simulink library "Library_Betriebsstrategie"  (R2018b)
settings: Solver=VariableStepAuto  StartTime=0.0  StopTime=10.0  RelTol=1e-3  EnableMultiTasking=on
undefined symbols (not defined in the file): akt_eUELG_HA, akt_eUELG_VA, akt_keinMVS_HA, akt_keinMVS_VA, akt_LSD_HA, akt_LSD_VA, akt_mUELG_HA, akt_mUELG_VA, akt_OD_HA, akt_OD_VA, DiscIntNeverNeededParam, magnitude, mu_road, mu_road_LF, mu_road_LR, mu_road_RF, mu_road_RR, par_MDT, par_VEH, stepsize
libraries: simulink x13
(part 3 of 6)

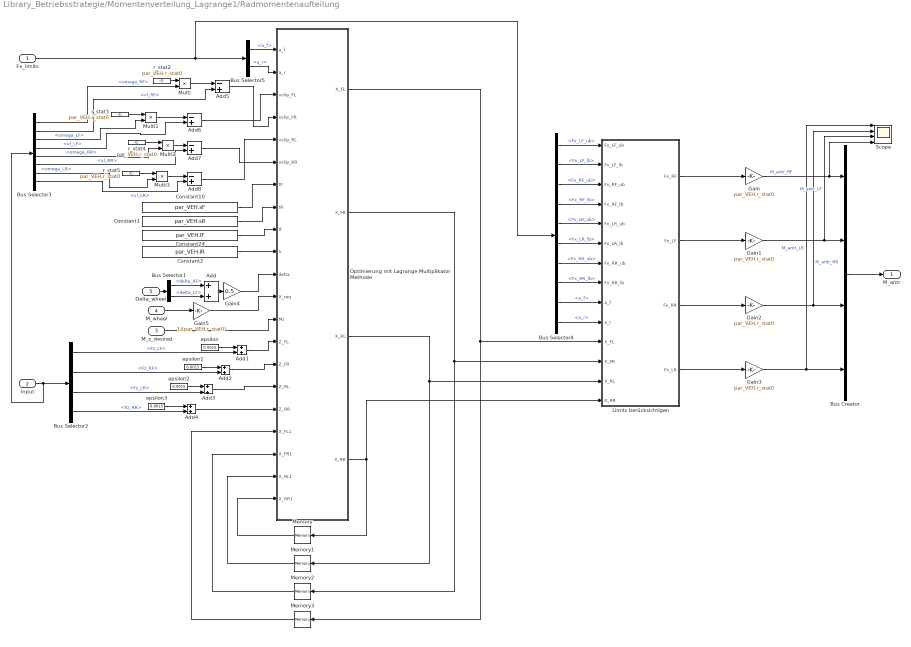
== system Library_Betriebsstrategie/Momentenverteilung_Lagrange1/Radmomentenaufteilung ==
  Fx_limits : Inport
  Input : Inport  Port=2
  M_z_desired : Inport  Port=3
  M_wheel : Inport  Port=4
  Delta_wheel : Inport  Port=5
  Add{,1..4} (5 alike) : Sum
  Add{5..8} (4 alike) : Sum  Inputs=-+
  Bus Creator : BusCreator  Inputs=4
  Bus Selector1 : BusSelector  OutputSignals=delta_RF,delta_LF
  Bus Selector2 : BusSelector  OutputSignals=Fz.Fz_LF,Fz.Fz_RF,Fz.Fz_LR,Fz.Fz_RR
  Bus Selector3 : BusSelector  OutputSignals=omega.omega_RF,vl.vl_RF,omega.omega_LF,vl.vl_LF,omega.omega_RR,vl.vl_RR,omega.omega_LR,vl.vl_LR
  Bus Selector4 : BusSelector  OutputSignals=Fx_LF_ub,Fx_LF_lb,Fx_RF_ub,Fx_RF_lb,Fx_LR_ub,Fx_LR_lb,Fx_RR_ub,Fx_RR_lb,a_f,a_r
  Bus Selector5 : BusSelector  OutputSignals=a_f,a_r
  Constant1 : Constant  Value=par_VEH.sR
  Constant10 : Constant  Value=par_VEH.sF
  Constant2 : Constant  Value=par_VEH.lR
  Constant24 : Constant  Value=par_VEH.lF
  Gain{,1..3} (4 alike) : Gain  Gain=par_VEH.r_stat0
  Gain4 : Gain  Gain=0.5
  Gain5 : Gain  Gain=1/(par_VEH.r_stat0)
  Limits berücksichtigen : MATLAB Function  TreatAsAtomicUnit=on
  Memory{,1..3} (4 alike) : Memory
  Multi{,1..3} (4 alike) : Product  Inputs=**
  Optimierung mit Lagrange Multiplikator Methode : MATLAB Function  TreatAsAtomicUnit=on
  Scope : Scope  NumInputPorts=4
  epsilon{,1..3} (4 alike) : Constant  Value=0.0015
  r_stat{2..5} (4 alike) : Constant  Value=par_VEH.r_stat0
  M_antr : Outport
  wires:
  Bus Selector5/2 -> Optimierung mit Lagrange Multiplikator Methode/2(a_r)  "<a_r>"
  Bus Selector5/1 -> Optimierung mit Lagrange Multiplikator Methode/1(a_f)  "<a_f>"
  Fx_limits/1 -> Bus Selector5/1, Bus Selector4/1
  Limits berücksichtigen/4(Fx_LR) -> Gain3/1
  Limits berücksichtigen/3(Fx_RR) -> Gain2/1
  Limits berücksichtigen/2(Fx_LF) -> Gain1/1
  Limits berücksichtigen/1(Fx_RF) -> Gain/1
  Optimierung mit Lagrange Multiplikator Methode/3(X_RL) -> Memory1/1, Limits berücksichtigen/13(X_RL)
  Bus Selector4/10 -> Limits berücksichtigen/10(a_r)  "<a_r>"
  Bus Selector4/9 -> Limits berücksichtigen/9(a_f)  "<a_f>"
  Bus Selector4/8 -> Limits berücksichtigen/8(Fx_RR_lb)  "<Fx_RR_lb>"
  Bus Selector4/7 -> Limits berücksichtigen/7(Fx_RR_ub)  "<Fx_RR_ub>"
  Bus Selector4/6 -> Limits berücksichtigen/6(Fx_LR_lb)  "<Fx_LR_lb>"
  Bus Selector4/5 -> Limits berücksichtigen/5(Fx_LR_ub)  "<Fx_LR_ub>"
  Bus Selector4/4 -> Limits berücksichtigen/4(Fx_RF_lb)  "<Fx_RF_lb>"
  Bus Selector4/3 -> Limits berücksichtigen/3(Fx_RF_ub)  "<Fx_RF_ub>"
  Bus Selector4/2 -> Limits berücksichtigen/2(Fx_LF_lb)  "<Fx_LF_lb>"
  Bus Selector4/1 -> Limits berücksichtigen/1(Fx_LF_ub)  "<Fx_LF_ub>"
  Memory1/1 -> Optimierung mit Lagrange Multiplikator Methode/20(X_RL1)
  Add3/1 -> Optimierung mit Lagrange Multiplikator Methode/16(Z_RL)
  Bus Creator/1 -> M_antr/1
  Gain/1 -> Scope/4, Bus Creator/1  "M_antr_RF"
  Gain1/1 -> Bus Creator/2, Scope/3  "M_antr_LF"
  Gain2/1 -> Bus Creator/3, Scope/2  "M_antr_RR"
  Gain3/1 -> Bus Creator/4, Scope/1  "M_antr_LR"
  Constant10/1 -> Optimierung mit Lagrange Multiplikator Methode/7(tF)
  Constant1/1 -> Optimierung mit Lagrange Multiplikator Methode/8(tR)
  Constant24/1 -> Optimierung mit Lagrange Multiplikator Methode/9(lf)
  Constant2/1 -> Optimierung mit Lagrange Multiplikator Methode/10(lr)
  Delta_wheel/1 -> Bus Selector1/1
  Bus Selector1/1 -> Add/1  "<delta_RF>"
  Bus Selector1/2 -> Add/2  "<delta_LF>"
  Add/1 -> Gain4/1
  Gain4/1 -> Optimierung mit Lagrange Multiplikator Methode/11(delta)
  M_z_desired/1 -> Optimierung mit Lagrange Multiplikator Methode/13(Mz)
  M_wheel/1 -> Gain5/1
  Gain5/1 -> Optimierung mit Lagrange Multiplikator Methode/12(X_req)
  Optimierung mit Lagrange Multiplikator Methode/1(X_FL) -> Memory3/1, Limits berücksichtigen/11(X_FL)
  Optimierung mit Lagrange Multiplikator Methode/2(X_FR) -> Memory2/1, Limits berücksichtigen/12(X_FR)
  Optimierung mit Lagrange Multiplikator Methode/4(X_RR) -> Memory/1, Limits berücksichtigen/14(X_RR)
  Memory/1 -> Optimierung mit Lagrange Multiplikator Methode/21(X_RR1)
  Memory2/1 -> Optimierung mit Lagrange Multiplikator Methode/19(X_FR1)
  Memory3/1 -> Optimierung mit Lagrange Multiplikator Methode/18(X_FL1)
  Add1/1 -> Optimierung mit Lagrange Multiplikator Methode/14(Z_FL)
  Bus Selector2/4 -> Add4/2  "<Fz_RR>"
  Bus Selector2/3 -> Add3/2  "<Fz_LR>"
  Bus Selector2/2 -> Add2/2  "<Fz_RF>"
  Bus Selector2/1 -> Add1/2  "<Fz_LF>"
  Add4/1 -> Optimierung mit Lagrange Multiplikator Methode/17(Z_RR)
  Add2/1 -> Optimierung mit Lagrange Multiplikator Methode/15(Z_FR)
  epsilon/1 -> Add1/1
  epsilon1/1 -> Add2/1
  epsilon2/1 -> Add3/1
  epsilon3/1 -> Add4/1
  Add7/1 -> Optimierung mit Lagrange Multiplikator Methode/6(vslip_RR)
  Add8/1 -> Optimierung mit Lagrange Multiplikator Methode/5(vslip_RL)
  Bus Selector3/8 -> Add8/2  "<vl_LR>"
  Bus Selector3/6 -> Add7/2  "<vl_RR>"
  Bus Selector3/4 -> Add6/2  "<vl_LF>"
  Bus Selector3/7 -> Multi3/2  "<omega_LR>"
  Bus Selector3/5 -> Multi2/2  "<omega_RR>"
  Bus Selector3/3 -> Multi1/2  "<omega_LF>"
  Multi2/1 -> Add7/1
  Multi3/1 -> Add8/1
  r_stat5/1 -> Multi3/1
  r_stat4/1 -> Multi2/1
  Multi1/1 -> Add6/1
  r_stat3/1 -> Multi1/1
  Bus Selector3/2 -> Add5/2  "<vl_RF>"
  Multi/1 -> Add5/1
  Bus Selector3/1 -> Multi/2  "<omega_RF>"
  Input/1 -> Bus Selector3/1, Bus Selector2/1
  Add5/1 -> Optimierung mit Lagrange Multiplikator Methode/4(vslip_FR)
  Add6/1 -> Optimierung mit Lagrange Multiplikator Methode/3(vslip_FL)
  r_stat2/1 -> Multi/1

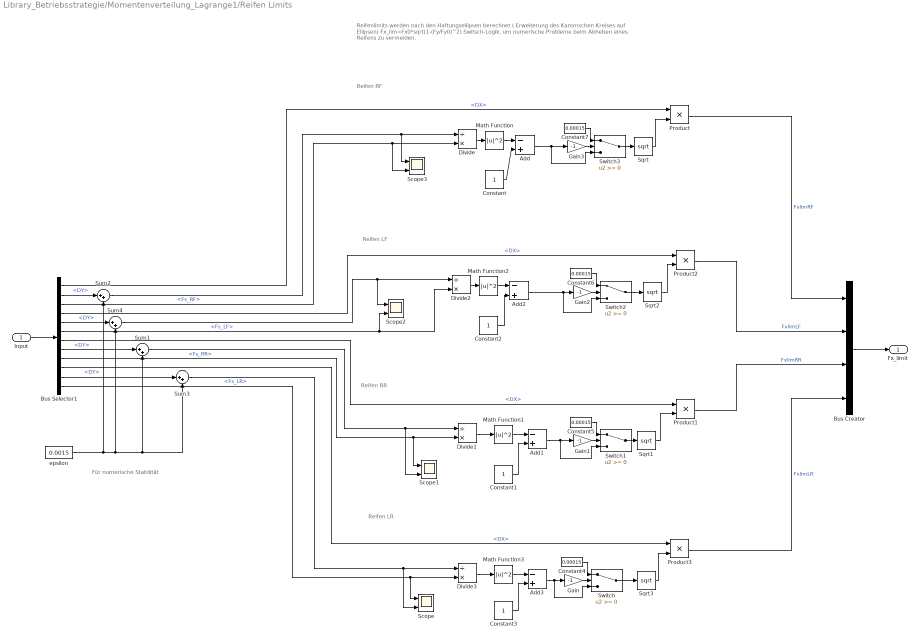
== system Library_Betriebsstrategie/Momentenverteilung_Lagrange1/Reifen Limits ==
  note: Reifen RF
  note: Reifen LF
  note: Reifen RR
  note: Reifen LR
  note: Für numerische Stabilität
  note: Reifenlimits werden nach den Haftungsellipsen berechnet ( Erweiterung des Kammschen Kreises auf Ellipsen)
      | Fx_lim=Fx0*sqrt(1-(Fy/Fy0)^2)
      |
      | Switsch-Logik, um numerische Probleme beim Abheben eines Reifens zu vermeiden.
  Input : Inport
  Add{,1..3} (4 alike) : Sum  Inputs=-+
  Bus Creator : BusCreator  Inputs=4
  Bus Selector1 : BusSelector  OutputSignals=F0.F0_RF.DX,F0.F0_RF.DY,Fs.Fs_RF,F0.F0_LF.DX,F0.F0_LF.DY,Fs.Fs_LF,F0.F0_RR.DX,F0.F0_RR.DY,Fs.Fs_RR,F0.F0_LR.DX,F0.F0_LR.DY,Fs.Fs_LR
  Constant{,1..3} (4 alike) : Constant
  Constant{4..7} (4 alike) : Constant  Value=0.00015
  Divide{,1..3} (4 alike) : Product  Inputs=/*
  Gain{,1..3} (4 alike) : Gain  Gain=-1
  Math Function{,1..3} (4 alike) : Math  Operator=magnitude^2  SaturateOnIntegerOverflow=on
  Product{,1..3} (4 alike) : Product
  Scope{,1..3} (4 alike) : Scope  NumInputPorts=2
  Sqrt{,1..3} (4 alike) : Sqrt  SaturateOnIntegerOverflow=on
  Sum{1..4} (4 alike) : Sum  Inputs=|++
  Switch{,1..3} (4 alike) : Switch
  epsilon : Constant  Value=0.0015
  Fx_limit : Outport
  wires:
  Bus Selector1/10 -> Product3/1  "<DX>"
  Bus Selector1/5 -> Sum4/1  "<DY>"
  Bus Selector1/8 -> Sum1/1  "<DY>"
  Bus Selector1/11 -> Sum3/1  "<DY>"
  Bus Selector1/2 -> Sum2/1  "<DY>"
  epsilon/1 -> Sum3/2, Sum1/2, Sum4/2, Sum2/2
  Bus Selector1/1 -> Product/1  "<DX>"
  Sum2/1 -> Divide/1, Scope3/1
  Math Function/1 -> Add/1
  Constant/1 -> Add/2
  Sqrt/1 -> Product/2
  Bus Selector1/7 -> Product1/1  "<DX>"
  Sum1/1 -> Divide1/1, Scope1/2
  Divide1/1 -> Math Function1/1
  Math Function1/1 -> Add1/1
  Constant1/1 -> Add1/2
  Sqrt1/1 -> Product1/2
  Bus Selector1/4 -> Product2/1  "<DX>"
  Sum4/1 -> Divide2/1, Scope2/1
  Divide2/1 -> Math Function2/1
  Math Function2/1 -> Add2/1
  Constant2/1 -> Add2/2
  Sqrt2/1 -> Product2/2
  Sum3/1 -> Divide3/1, Scope/2
  Divide3/1 -> Math Function3/1
  Math Function3/1 -> Add3/1
  Constant3/1 -> Add3/2
  Sqrt3/1 -> Product3/2
  Divide/1 -> Math Function/1
  Input/1 -> Bus Selector1/1
  Bus Selector1/3 -> Divide/2, Scope3/2  "<Fs_RF>"
  Bus Selector1/6 -> Divide2/2, Scope2/2  "<Fs_LF>"
  Bus Selector1/9 -> Divide1/2, Scope1/1  "<Fs_RR>"
  Bus Selector1/12 -> Divide3/2, Scope/1  "<Fs_LR>"
  Product/1 -> Bus Creator/1  "FxlimRF"
  Product2/1 -> Bus Creator/2  "FxlimLF"
  Product1/1 -> Bus Creator/3  "FxlimRR"
  Product3/1 -> Bus Creator/4  "FxlimLR"
  Bus Creator/1 -> Fx_limit/1
  Add3/1 -> Switch/3, Gain/1
  Gain/1 -> Switch/2
  Constant4/1 -> Switch/1
  Switch/1 -> Sqrt3/1
  Add1/1 -> Gain1/1, Switch1/3
  Gain1/1 -> Switch1/2
  Constant5/1 -> Switch1/1
  Switch1/1 -> Sqrt1/1
  Add2/1 -> Switch2/3, Gain2/1
  Gain2/1 -> Switch2/2
  Constant6/1 -> Switch2/1
  Switch2/1 -> Sqrt2/1
  Add/1 -> Gain3/1, Switch3/3
  Gain3/1 -> Switch3/2
  Constant7/1 -> Switch3/1
  Switch3/1 -> Sqrt/1

== system Library_Betriebsstrategie/Momentenverteilung_Lagrange2/Feedback Controller ==
  note: 1/2 sigma(Tc)
  note: M_z punkt = - Iz * K * sign(sigma - 1/2sigma(Tc))
  note: Sigmoid Funktion
  Input : Inport
  Gierrate ref : Inport  Port=2
  -1 : Gain  Gain=-1
  Abs : Abs
  Add : Sum
  Bus Selector2 : BusSelector  OutputSignals=psi.psip
  Constant1 : Constant  Value=par_VEH.Iz
  Discrete D : simulink/Discrete/Discrete Derivative  gainval=1.0  ICPrevScaledInput=0.0  OutMin=[]  OutMax=[]  OutDataType=fixdt(1, 16)  OutScaling=2^-10  DoSatur=off
  Discrete-Time Integrator : DiscreteIntegrator  SampleTime=-1  LimitOutput=on  UpperSaturationLimit=par_VEH.Iz/10  LowerSaturationLimit=-par_VEH.Iz/10  ICPrevOutput=DiscIntNeverNeededParam  ICPrevScaledInput=DiscIntNeverNeededParam
  Divide : Product  Inputs=*/
  Divide1 : Product  Inputs=*/
  Einheitenkorrektur : Constant  Value=1000
  Gain : Gain  Gain=0.5
  K : Gain  Gain=8
  Memory : Memory  LinearizeAsDelay=on
  Product : Product
  Scope : Scope  NumInputPorts=2
  Sum : Sum  Inputs=|-+
  Sum1 : Sum  Inputs=|+-
  Unit Delay : UnitDelay  SampleTime=-1
  Zero Crossing : Subsystem
  epsilon : Constant  Value=0.015
  M_z_desired : Outport
  wires:
  Gierrate ref/1 -> Scope/1, Sum/1
  Sum/1 -> Sum1/1, Zero Crossing/3(e0), Discrete D/1  "sigma = - error"
  Sum1/1 -> Divide/1, Abs/1
  Abs/1 -> Add/1
  epsilon/1 -> Add/2
  Add/1 -> Divide/2
  Divide/1 -> K/1
  K/1 -> Product/1
  Product/1 -> -1/1
  -1/1 -> Discrete-Time Integrator/1
  Discrete-Time Integrator/1 -> M_z_desired/1
  Discrete D/1 -> Zero Crossing/1(de0), Unit Delay/1
  Gain/1 -> Sum1/2
  Memory/1 -> Zero Crossing/4(e1)
  Unit Delay/1 -> Zero Crossing/2(de1)
  Zero Crossing/1(error(Tc)) -> Memory/1, Gain/1
  Einheitenkorrektur/1 -> Divide1/2
  Divide1/1 -> Product/2
  Input/1 -> Bus Selector2/1
  Bus Selector2/1 -> Scope/2, Sum/2  "<psip>"
  Constant1/1 -> Divide1/1

== system Library_Betriebsstrategie/Momentenverteilung_Lagrange2/Gierrate Referenz Berechnung ==
  note: Gewünschte Gierrate nach:
      | psip_desired = vx * delta / (l + vx^2 * K_us )
  note: Limit für die Gierrate
  input : Inport
  delta_wheel : Inport  Port=2
  2 Räder : Constant  Value=0.5
  Abs : Abs
  Abs1 : Abs
  Add : Sum
  Add1 : Sum  Inputs=+--
  Add2 : Sum
  Bus Selector1 : BusSelector  OutputSignals=delta_RF,delta_LF
  Bus Selector2 : BusSelector  OutputSignals=x.ax,beta.beta,beta.betap,x.vx
  Constant1 : Constant  Value=par_VEH.g
  Constant10 : Constant  Value=par_VEH.l
  Constant20 : Constant  Value=0.25*(mu_road_RF+mu_road_RR+mu_road_LF+mu_road_LR)
  Divide : Product  Inputs=*/
  Divide1 : Product  Inputs=**/
  Divide2 : Product  Inputs=**/
  Divide3 : Product  Inputs=*/
  Kus : Constant  Value=0
  Product : Product
  Product1 : Product
  Product2 : Product
  Scope : Scope  NumInputPorts=2
  Sicherheitsfaktor : Gain  Gain=0.90
  Sign : Signum
  Sqrt : Sqrt  SaturateOnIntegerOverflow=on
  Sum : Sum  Inputs=|++
  Sum1 : Sum  Inputs=|++
  delta mittel : Product
  eins : Constant
  epsilon : Constant  Value=0.0015
  min : MinMax  Inputs=2
  tan (beta)1 : Trigonometry  Operator=tan
  tan^2 (beta)1 : Math  Operator=square  SaturateOnIntegerOverflow=on
  vx^2 : Math  Operator=square  SaturateOnIntegerOverflow=on
  Gierrate ref : Outport
  wires:
  Product/1 -> Divide/1
  Constant10/1 -> Sum/2
  vx^2/1 -> Product1/1
  Sum/1 -> Divide/2
  Product1/1 -> Sum/1
  Kus/1 -> Product1/2
  Divide/1 -> Abs/1  "Gierrate gewuenscht"
  delta_wheel/1 -> Bus Selector1/1
  Bus Selector1/1 -> Add/1  "<delta_RF>"
  Bus Selector1/2 -> Add/2  "<delta_LF>"
  Add/1 -> Scope/2, delta mittel/1
  2 Räder/1 -> delta mittel/2
  delta mittel/1 -> Sign/1, Product/2
  input/1 -> Bus Selector2/1
  Bus Selector2/4 -> Sum1/1, vx^2/1, Product/1  "<vx>"
  Sicherheitsfaktor/1 -> Abs1/1  "Gierrate Limit"
  Add1/1 -> Sicherheitsfaktor/1
  Sign/1 -> Product2/1  "Vorzeichen von delta"
  min/1 -> Product2/2
  Product2/1 -> Scope/1, Gierrate ref/1
  Abs/1 -> min/1
  Abs1/1 -> min/2
  Divide1/1 -> Add1/1
  Constant1/1 -> Divide1/2
  Constant20/1 -> Divide1/1
  Divide2/1 -> Add1/2
  Bus Selector2/1 -> Divide2/2  "<ax>"
  tan (beta)1/1 -> tan^2 (beta)1/1, Divide2/1
  Bus Selector2/2 -> tan (beta)1/1  "<beta>"
  Divide3/1 -> Add1/3
  Bus Selector2/3 -> Divide3/1  "<betap>"
  tan^2 (beta)1/1 -> Add2/1
  eins/1 -> Add2/2
  Add2/1 -> Sqrt/1
  Sqrt/1 -> Divide3/2
  Sum1/1 -> Divide2/3, Divide1/3
  epsilon/1 -> Sum1/2

== system Library_Betriebsstrategie/Momentenverteilung_Lagrange2/Limitierungen gesamt (mit MVS Limits) ==
  Fx_limit : Inport
  M_limit : Inport  Port=2
  M_limit_zentral : Inport  Port=3
  Aktuatoren und Delta TV : Subsystem
  Bus Creator : BusCreator  Inputs=10
  Bus Selector : BusSelector  OutputSignals=FxlimRF,FxlimLF,FxlimRR,FxlimLR
  Bus Selector1 : BusSelector  OutputSignals=M_RF_ub,M_RF_lb,M_LF_ub,M_LF_lb,M_RR_ub,M_RR_lb,M_LR_ub,M_LR_lb
  Bus Selector2 : BusSelector  OutputSignals=M_F_lb,M_F_ub,M_R_lb,M_R_ub
  Limits Zusammenführung : MATLAB Function  TreatAsAtomicUnit=on
  Scope : Scope  NumInputPorts=4
  Scope1 : Scope  NumInputPorts=4
  Scope2 : Scope  NumInputPorts=4
  r_stat0 : Constant  Value=par_VEH.r_stat0
  Fx_limits : Outport
  wires:
  Limits Zusammenführung/8(Fx_RR_lb) -> Bus Creator/8  "Fx_RR_lb"
  Limits Zusammenführung/7(Fx_RR_ub) -> Bus Creator/7  "Fx_RR_ub"
  Limits Zusammenführung/6(Fx_LR_lb) -> Bus Creator/6  "Fx_LR_lb"
  Limits Zusammenführung/5(Fx_LR_ub) -> Bus Creator/5  "Fx_LR_ub"
  Limits Zusammenführung/4(Fx_RF_lb) -> Bus Creator/4, Scope1/1  "Fx_RF_lb"
  Limits Zusammenführung/3(Fx_RF_ub) -> Bus Creator/3, Scope1/2  "Fx_RF_ub"
  Limits Zusammenführung/2(Fx_LF_lb) -> Bus Creator/2, Scope1/3  "Fx_LF_lb"
  Limits Zusammenführung/1(Fx_LF_ub) -> Bus Creator/1, Scope1/4  "Fx_LF_ub"
  Aktuatoren und Delta TV/2(Delta_T_r) -> Scope2/2, Limits Zusammenführung/18(DELTA_T_r)
  Aktuatoren und Delta TV/1(Delta_T_f) -> Scope2/1, Limits Zusammenführung/17(DELTA_T_f)
  r_stat0/1 -> Limits Zusammenführung/21(r)
  Fx_limit/1 -> Bus Selector/1
  M_limit/1 -> Bus Selector1/1
  Bus Creator/1 -> Fx_limits/1
  Bus Selector/1 -> Limits Zusammenführung/1(FxlimRF), Scope/4  "<FxlimRF>"
  Bus Selector/2 -> Limits Zusammenführung/2(FxlimLF), Scope/3  "<FxlimLF>"
  Bus Selector/3 -> Scope/2, Limits Zusammenführung/3(FxlimRR)  "<FxlimRR>"
  Bus Selector/4 -> Limits Zusammenführung/4(FxlimLR), Scope/1  "<FxlimLR>"
  Bus Selector1/1 -> Limits Zusammenführung/5(M_RF_ub)  "<M_RF_ub>"
  Bus Selector1/2 -> Limits Zusammenführung/6(M_RF_lb)  "<M_RF_lb>"
  Bus Selector1/3 -> Limits Zusammenführung/7(M_LF_ub)  "<M_LF_ub>"
  Bus Selector1/4 -> Limits Zusammenführung/8(M_LF_lb)  "<M_LF_lb>"
  Bus Selector1/5 -> Limits Zusammenführung/9(M_RR_ub)  "<M_RR_ub>"
  Bus Selector1/6 -> Limits Zusammenführung/10(M_RR_lb)  "<M_RR_lb>"
  Bus Selector1/7 -> Limits Zusammenführung/11(M_LR_ub)  "<M_LR_ub>"
  Bus Selector1/8 -> Limits Zusammenführung/12(M_LR_lb)  "<M_LR_lb>"
  M_limit_zentral/1 -> Bus Selector2/1
  Bus Selector2/1 -> Limits Zusammenführung/13(M_F_lb)  "<M_F_lb>"
  Bus Selector2/2 -> Limits Zusammenführung/14(M_F_ub)  "<M_F_ub>"
  Bus Selector2/3 -> Limits Zusammenführung/15(M_R_lb)  "<M_R_lb>"
  Bus Selector2/4 -> Limits Zusammenführung/16(M_R_ub)  "<M_R_ub>"
  Aktuatoren und Delta TV/3(A_f) -> Scope2/3, Bus Creator/9, Limits Zusammenführung/19(a_f)
  Aktuatoren und Delta TV/4(A_r) -> Scope2/4, Bus Creator/10, Limits Zusammenführung/20(a_r)

== system Library_Betriebsstrategie/Momentenverteilung_Lagrange2/Momente für die Reibbremse ==
  M_antr : Inport
  M_wheel : Inport  Port=2
  v_x : Inport  Port=3
  Add : Sum  Inputs=-+
  Add1 : Sum  Inputs=++++
  Bias : Bias  Bias=-1
  Bus Creator1 : BusCreator  Inputs=4
  Bus Selector : BusSelector  OutputSignals=M_antr_LF,M_antr_LR,M_antr_RF,M_antr_RR
  Constant1 : Constant  Value=par_VEH.bkv
  Product4 : Product  Inputs=3
  Product5 : Product  Inputs=3
  Saturation2 : Saturate  UpperLimit=0  LowerLimit=-5000
  Sign : Signum
  Signal Conversion : SignalConversion  OverrideOpt=off
  Signal Conversion1 : SignalConversion  OverrideOpt=off
  Unary Minus : UnaryMinus
  Unit Delay2 : UnitDelay  InitialCondition=2  SampleTime=-1
  M_brems : Outport
  wires:
  Add/1 -> Saturation2/1
  Saturation2/1 -> Product5/1, Product4/2
  Bias/1 -> Unary Minus/1
  Unary Minus/1 -> Product5/2
  Sign/1 -> Product4/3, Product5/3
  Unit Delay2/1 -> Sign/1
  Constant1/1 -> Product4/1, Bias/1
  v_x/1 -> Unit Delay2/1
  M_wheel/1 -> Add/2
  M_antr/1 -> Bus Selector/1
  Bus Selector/4 -> Add1/4  "<M_antr_RR>"
  Bus Selector/3 -> Add1/3  "<M_antr_RF>"
  Bus Selector/2 -> Add1/2  "<M_antr_LR>"
  Bus Selector/1 -> Add1/1  "<M_antr_LF>"
  Add1/1 -> Add/1
  Bus Creator1/1 -> M_brems/1
  Product4/1 -> Bus Creator1/1, Signal Conversion/1  "M_brems_LF"
  Signal Conversion/1 -> Bus Creator1/2  "M_brems_LR"
  Product5/1 -> Signal Conversion1/1, Bus Creator1/3  "M_brems_RF"
  Signal Conversion1/1 -> Bus Creator1/4  "M_brems_RR"

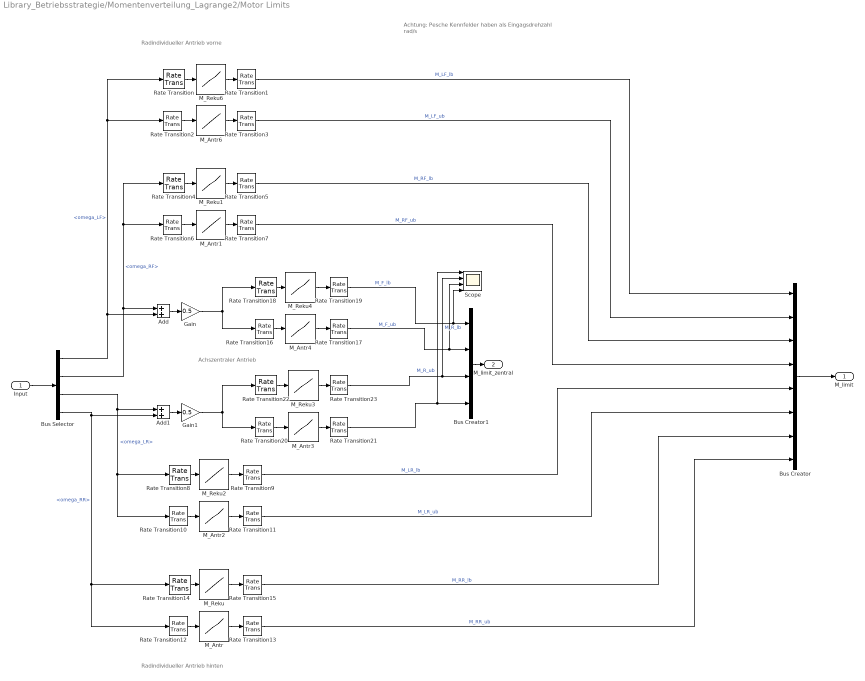
== system Library_Betriebsstrategie/Momentenverteilung_Lagrange2/Motor Limits ==
  note: Achszentraler Antrieb
  note: Radindividueller Antrieb hinten
  note: Radindividueller Antrieb vorne
  note: Achtung:
      | Pesche Kennfelder haben als Eingagsdrehzahl rad/s
  Input : Inport
  Add : Sum
  Add1 : Sum
  Bus Creator : BusCreator  Inputs=8
  Bus Creator1 : BusCreator  Inputs=4
  Bus Selector : BusSelector  OutputSignals=omega.omega_LF,omega.omega_RF,omega.omega_LR,omega.omega_RR
  Gain : Gain  Gain=0.5
  Gain1 : Gain  Gain=0.5
  M_Antr : Lookup_n-D  NumberOfTableDimensions=1  BreakpointsForDimension1=par_MDT.HA.em.MaxMotorTrqCurve_w/par_MDT.HA.trans.i_gears(1)  Table=par_MDT.HA.em.MaxMotorTrqCurve_M*par_MDT.HA.trans.i_gears(1)  ExtrapMethod=Clip  UseLastTableValue=on  InternalRulePriority=Speed  RndMeth=Simplest  InputSameDT=on
  M_Antr1 : Lookup_n-D  NumberOfTableDimensions=1  BreakpointsForDimension1=par_MDT.VA.em.MaxMotorTrqCurve_w/par_MDT.VA.trans.i_gears(1)  Table=par_MDT.VA.em.MaxMotorTrqCurve_M*par_MDT.VA.trans.i_gears(1)  ExtrapMethod=Clip  UseLastTableValue=on  InternalRulePriority=Speed  RndMeth=Simplest  InputSameDT=on
  M_Antr2 : Lookup_n-D  NumberOfTableDimensions=1  BreakpointsForDimension1=par_MDT.HA.em.MaxMotorTrqCurve_w/par_MDT.HA.trans.i_gears(1)  Table=par_MDT.HA.em.MaxMotorTrqCurve_M*par_MDT.HA.trans.i_gears(1)  ExtrapMethod=Clip  UseLastTableValue=on  InternalRulePriority=Speed  RndMeth=Simplest  InputSameDT=on
  M_Antr3 : Lookup_n-D  NumberOfTableDimensions=1  BreakpointsForDimension1=par_MDT.HA.em.MaxMotorTrqCurve_w/par_MDT.HA.trans.i_gears(1)  Table=par_MDT.HA.em.MaxMotorTrqCurve_M*par_MDT.HA.trans.i_gears(1)  ExtrapMethod=Clip  UseLastTableValue=on  InternalRulePriority=Speed  RndMeth=Simplest  InputSameDT=on
  M_Antr4 : Lookup_n-D  NumberOfTableDimensions=1  BreakpointsForDimension1=par_MDT.VA.em.MaxMotorTrqCurve_w/par_MDT.VA.trans.i_gears(1)  Table=par_MDT.VA.em.MaxMotorTrqCurve_M*par_MDT.VA.trans.i_gears(1)  ExtrapMethod=Clip  UseLastTableValue=on  InternalRulePriority=Speed  RndMeth=Simplest  InputSameDT=on
  M_Antr6 : Lookup_n-D  NumberOfTableDimensions=1  BreakpointsForDimension1=par_MDT.VA.em.MaxMotorTrqCurve_w/par_MDT.VA.trans.i_gears(1)  Table=par_MDT.VA.em.MaxMotorTrqCurve_M*par_MDT.VA.trans.i_gears(1)  ExtrapMethod=Clip  UseLastTableValue=on  InternalRulePriority=Speed  RndMeth=Simplest  InputSameDT=on
  M_Reku : Lookup_n-D  NumberOfTableDimensions=1  BreakpointsForDimension1=par_MDT.HA.em.MaxGeneratorTrqCurve_w/par_MDT.HA.trans.i_gears(1)  Table=par_MDT.HA.em.MaxGeneratorTrqCurve_M*par_MDT.HA.trans.i_gears(1)  ExtrapMethod=Clip  UseLastTableValue=on  InternalRulePriority=Speed  RndMeth=Simplest  InputSameDT=on
  M_Reku1 : Lookup_n-D  NumberOfTableDimensions=1  BreakpointsForDimension1=par_MDT.VA.em.MaxGeneratorTrqCurve_w/par_MDT.VA.trans.i_gears(1)  Table=par_MDT.VA.em.MaxGeneratorTrqCurve_M*par_MDT.VA.trans.i_gears(1)  ExtrapMethod=Clip  UseLastTableValue=on  InternalRulePriority=Speed  RndMeth=Simplest  InputSameDT=on
  M_Reku2 : Lookup_n-D  NumberOfTableDimensions=1  BreakpointsForDimension1=par_MDT.HA.em.MaxGeneratorTrqCurve_w/par_MDT.HA.trans.i_gears(1)  Table=par_MDT.HA.em.MaxGeneratorTrqCurve_M*par_MDT.HA.trans.i_gears(1)  ExtrapMethod=Clip  UseLastTableValue=on  InternalRulePriority=Speed  RndMeth=Simplest  InputSameDT=on
  M_Reku3 : Lookup_n-D  NumberOfTableDimensions=1  BreakpointsForDimension1=par_MDT.HA.em.MaxGeneratorTrqCurve_w/par_MDT.HA.trans.i_gears(1)  Table=par_MDT.HA.em.MaxGeneratorTrqCurve_M*par_MDT.HA.trans.i_gears(1)  ExtrapMethod=Clip  UseLastTableValue=on  InternalRulePriority=Speed  RndMeth=Simplest  InputSameDT=on
  M_Reku4 : Lookup_n-D  NumberOfTableDimensions=1  BreakpointsForDimension1=par_MDT.VA.em.MaxGeneratorTrqCurve_w/par_MDT.VA.trans.i_gears(1)  Table=par_MDT.VA.em.MaxGeneratorTrqCurve_M*par_MDT.VA.trans.i_gears(1)  ExtrapMethod=Clip  UseLastTableValue=on  InternalRulePriority=Speed  RndMeth=Simplest  InputSameDT=on
  M_Reku6 : Lookup_n-D  NumberOfTableDimensions=1  BreakpointsForDimension1=par_MDT.VA.em.MaxGeneratorTrqCurve_w/par_MDT.VA.trans.i_gears(1)  Table=par_MDT.VA.em.MaxGeneratorTrqCurve_M*par_MDT.VA.trans.i_gears(1)  ExtrapMethod=Clip  UseLastTableValue=on  InternalRulePriority=Speed  RndMeth=Simplest  InputSameDT=on
  Rate Transition{,2,4,6,8,10,12,14,16,18,20,22} (12 alike) : RateTransition  OutPortSampleTime=stepsize*10
  Rate Transition{1,3,5,7,9,11,13,15,17,19,21,23} (12 alike) : RateTransition  OutPortSampleTimeOpt=Inherit  OutPortSampleTime=0.001
  Scope : Scope  NumInputPorts=4
  M_limit : Outport
  M_limit_zentral : Outport  Port=2
  wires:
  Rate Transition17/1 -> Bus Creator1/2, Scope/3  "M_F_ub"
  Bus Creator1/1 -> M_limit_zentral/1
  Bus Creator/1 -> M_limit/1
  Rate Transition13/1 -> Bus Creator/8  "M_RR_ub"
  Rate Transition15/1 -> Bus Creator/7  "M_RR_lb"
  Rate Transition11/1 -> Bus Creator/6  "M_LR_ub"
  Rate Transition9/1 -> Bus Creator/5  "M_LR_lb"
  Rate Transition1/1 -> Bus Creator/1  "M_LF_lb"
  Rate Transition7/1 -> Bus Creator/4  "M_RF_ub"
  Rate Transition5/1 -> Bus Creator/3  "M_RF_lb"
  Rate Transition3/1 -> Bus Creator/2  "M_LF_ub"
  Input/1 -> Bus Selector/1
  Rate Transition2/1 -> M_Antr6/1
  M_Antr6/1 -> Rate Transition3/1
  M_Reku6/1 -> Rate Transition1/1
  Bus Selector/1 -> Add/2, Rate Transition2/1, Rate Transition/1  "<omega_LF>"
  Rate Transition6/1 -> M_Antr1/1
  M_Antr1/1 -> Rate Transition7/1
  Rate Transition4/1 -> M_Reku1/1
  M_Reku1/1 -> Rate Transition5/1
  Bus Selector/2 -> Rate Transition6/1, Rate Transition4/1, Add/1  "<omega_RF>"
  Rate Transition10/1 -> M_Antr2/1
  M_Antr2/1 -> Rate Transition11/1
  Rate Transition8/1 -> M_Reku2/1
  M_Reku2/1 -> Rate Transition9/1
  Rate Transition12/1 -> M_Antr/1
  M_Antr/1 -> Rate Transition13/1
  Rate Transition14/1 -> M_Reku/1
  M_Reku/1 -> Rate Transition15/1
  Bus Selector/3 -> Add1/1, Rate Transition8/1, Rate Transition10/1  "<omega_LR>"
  Bus Selector/4 -> Add1/2, Rate Transition12/1, Rate Transition14/1  "<omega_RR>"
  Rate Transition16/1 -> M_Antr4/1
  M_Antr4/1 -> Rate Transition17/1
  Rate Transition18/1 -> M_Reku4/1
  M_Reku4/1 -> Rate Transition19/1
  Rate Transition20/1 -> M_Antr3/1
  M_Antr3/1 -> Rate Transition21/1
  Rate Transition22/1 -> M_Reku3/1
  M_Reku3/1 -> Rate Transition23/1
  Add/1 -> Gain/1
  Gain/1 -> Rate Transition16/1, Rate Transition18/1
  Add1/1 -> Gain1/1
  Gain1/1 -> Rate Transition20/1, Rate Transition22/1
  Rate Transition19/1 -> Bus Creator1/1, Scope/4  "M_F_lb"
  Rate Transition23/1 -> Bus Creator1/3, Scope/2  "M_R_lb"
  Rate Transition21/1 -> Bus Creator1/4, Scope/1  "M_R_ub"
  Rate Transition/1 -> M_Reku6/1

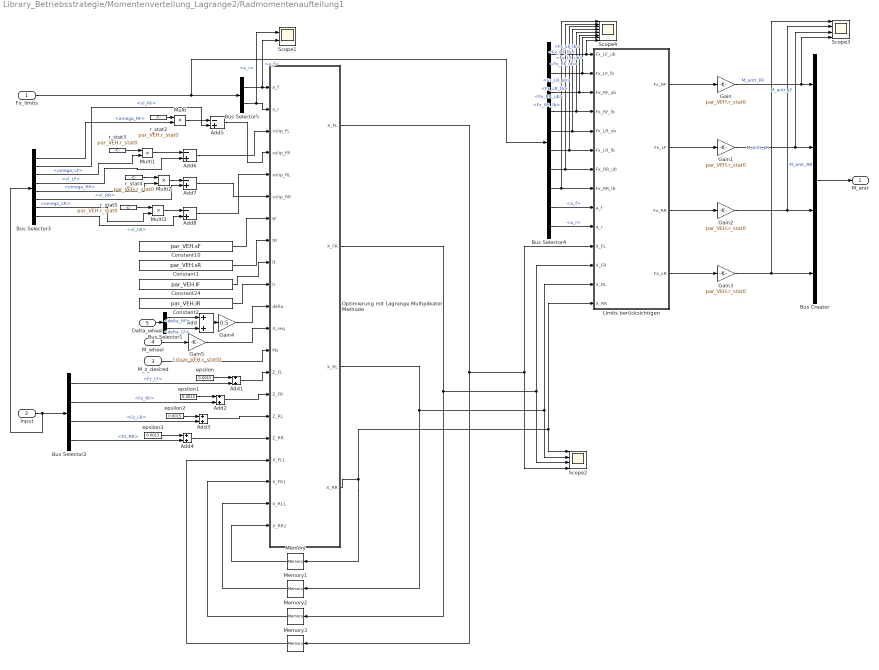
== system Library_Betriebsstrategie/Momentenverteilung_Lagrange2/Radmomentenaufteilung1 ==
  Fx_limits : Inport
  Input : Inport  Port=2
  M_z_desired : Inport  Port=3
  M_wheel : Inport  Port=4
  Delta_wheel : Inport  Port=5
  Add{,1..4} (5 alike) : Sum
  Add{5..8} (4 alike) : Sum  Inputs=-+
  Bus Creator : BusCreator  Inputs=4
  Bus Selector1 : BusSelector  OutputSignals=delta_RF,delta_LF
  Bus Selector2 : BusSelector  OutputSignals=Fz.Fz_LF,Fz.Fz_RF,Fz.Fz_LR,Fz.Fz_RR
  Bus Selector3 : BusSelector  OutputSignals=omega.omega_RF,vl.vl_RF,omega.omega_LF,vl.vl_LF,omega.omega_RR,vl.vl_RR,omega.omega_LR,vl.vl_LR
  Bus Selector4 : BusSelector  OutputSignals=Fx_LF_ub,Fx_LF_lb,Fx_RF_ub,Fx_RF_lb,Fx_LR_ub,Fx_LR_lb,Fx_RR_ub,Fx_RR_lb,a_f,a_r
  Bus Selector5 : BusSelector  OutputSignals=a_f,a_r
  Constant1 : Constant  Value=par_VEH.sR
  Constant10 : Constant  Value=par_VEH.sF
  Constant2 : Constant  Value=par_VEH.lR
  Constant24 : Constant  Value=par_VEH.lF
  Gain{,1..3} (4 alike) : Gain  Gain=par_VEH.r_stat0
  Gain4 : Gain  Gain=0.5
  Gain5 : Gain  Gain=1/(par_VEH.r_stat0)
  Limits berücksichtigen : MATLAB Function  TreatAsAtomicUnit=on
  Memory{,1..3} (4 alike) : Memory
  Multi{,1..3} (4 alike) : Product  Inputs=**
  Optimierung mit Lagrange Multiplikator Methode : MATLAB Function  TreatAsAtomicUnit=on
  Scope1 : Scope  NumInputPorts=2
  Scope2 : Scope  NumInputPorts=4
  Scope3 : Scope  NumInputPorts=4
  Scope4 : Scope  NumInputPorts=8
  epsilon{,1..3} (4 alike) : Constant  Value=0.0015
  r_stat{2..5} (4 alike) : Constant  Value=par_VEH.r_stat0
  M_antr : Outport
  wires:
  Limits berücksichtigen/4(Fx_LR) -> Gain3/1
  Limits berücksichtigen/3(Fx_RR) -> Gain2/1
  Limits berücksichtigen/2(Fx_LF) -> Gain1/1
  Limits berücksichtigen/1(Fx_RF) -> Gain/1
  Bus Selector5/2 -> Scope1/1, Optimierung mit Lagrange Multiplikator Methode/2(a_r)  "<a_r>"
  Bus Selector5/1 -> Scope1/2, Optimierung mit Lagrange Multiplikator Methode/1(a_f)  "<a_f>"
  Fx_limits/1 -> Bus Selector5/1, Bus Selector4/1
  Optimierung mit Lagrange Multiplikator Methode/3(X_RL) -> Memory1/1, Scope2/2, Limits berücksichtigen/13(X_RL)
  Bus Selector4/10 -> Limits berücksichtigen/10(a_r)  "<a_r>"
  Bus Selector4/9 -> Limits berücksichtigen/9(a_f)  "<a_f>"
  Bus Selector4/8 -> Limits berücksichtigen/8(Fx_RR_lb), Scope4/1  "<Fx_RR_lb>"
  Bus Selector4/7 -> Limits berücksichtigen/7(Fx_RR_ub), Scope4/2  "<Fx_RR_ub>"
  Bus Selector4/6 -> Limits berücksichtigen/6(Fx_LR_lb), Scope4/3  "<Fx_LR_lb>"
  Bus Selector4/5 -> Limits berücksichtigen/5(Fx_LR_ub), Scope4/4  "<Fx_LR_ub>"
  Bus Selector4/4 -> Limits berücksichtigen/4(Fx_RF_lb), Scope4/5  "<Fx_RF_lb>"
  Bus Selector4/3 -> Limits berücksichtigen/3(Fx_RF_ub), Scope4/6  "<Fx_RF_ub>"
  Bus Selector4/2 -> Limits berücksichtigen/2(Fx_LF_lb), Scope4/7  "<Fx_LF_lb>"
  Bus Selector4/1 -> Limits berücksichtigen/1(Fx_LF_ub), Scope4/8  "<Fx_LF_ub>"
  Memory1/1 -> Optimierung mit Lagrange Multiplikator Methode/20(X_RL1)
  Add3/1 -> Optimierung mit Lagrange Multiplikator Methode/16(Z_RL)
  Bus Creator/1 -> M_antr/1
  Gain/1 -> Bus Creator/1, Scope3/4  "M_antr_RF"
  Gain1/1 -> Bus Creator/2, Scope3/3  "M_antr_LF"
  Gain2/1 -> Scope3/2, Bus Creator/3  "M_antr_RR"
  Gain3/1 -> Bus Creator/4, Scope3/1  "M_antr_LR"
  Constant10/1 -> Optimierung mit Lagrange Multiplikator Methode/7(tF)
  Constant1/1 -> Optimierung mit Lagrange Multiplikator Methode/8(tR)
  Constant24/1 -> Optimierung mit Lagrange Multiplikator Methode/9(lf)
  Constant2/1 -> Optimierung mit Lagrange Multiplikator Methode/10(lr)
  Delta_wheel/1 -> Bus Selector1/1
  Bus Selector1/1 -> Add/1  "<delta_RF>"
  Bus Selector1/2 -> Add/2  "<delta_LF>"
  Add/1 -> Gain4/1
  Gain4/1 -> Optimierung mit Lagrange Multiplikator Methode/11(delta)
  M_z_desired/1 -> Optimierung mit Lagrange Multiplikator Methode/13(Mz)
  M_wheel/1 -> Gain5/1
  Gain5/1 -> Optimierung mit Lagrange Multiplikator Methode/12(X_req)
  Optimierung mit Lagrange Multiplikator Methode/2(X_FR) -> Memory2/1, Scope2/3, Limits berücksichtigen/12(X_FR)
  Optimierung mit Lagrange Multiplikator Methode/4(X_RR) -> Scope2/1, Limits berücksichtigen/14(X_RR), Memory/1
  Memory/1 -> Optimierung mit Lagrange Multiplikator Methode/21(X_RR1)
  Memory2/1 -> Optimierung mit Lagrange Multiplikator Methode/19(X_FR1)
  Memory3/1 -> Optimierung mit Lagrange Multiplikator Methode/18(X_FL1)
  Add1/1 -> Optimierung mit Lagrange Multiplikator Methode/14(Z_FL)
  Bus Selector2/4 -> Add4/2  "<Fz_RR>"
  Bus Selector2/3 -> Add3/2  "<Fz_LR>"
  Bus Selector2/2 -> Add2/2  "<Fz_RF>"
  Bus Selector2/1 -> Add1/2  "<Fz_LF>"
  Add4/1 -> Optimierung mit Lagrange Multiplikator Methode/17(Z_RR)
  Add2/1 -> Optimierung mit Lagrange Multiplikator Methode/15(Z_FR)
  epsilon/1 -> Add1/1
  epsilon1/1 -> Add2/1
  epsilon2/1 -> Add3/1
  epsilon3/1 -> Add4/1
  Add7/1 -> Optimierung mit Lagrange Multiplikator Methode/6(vslip_RR)
  Add8/1 -> Optimierung mit Lagrange Multiplikator Methode/5(vslip_RL)
  Bus Selector3/8 -> Add8/2  "<vl_LR>"
  Bus Selector3/6 -> Add7/2  "<vl_RR>"
  Bus Selector3/4 -> Add6/2  "<vl_LF>"
  Bus Selector3/7 -> Multi3/2  "<omega_LR>"
  Bus Selector3/5 -> Multi2/2  "<omega_RR>"
  Bus Selector3/3 -> Multi1/2  "<omega_LF>"
  Multi2/1 -> Add7/1
  Multi3/1 -> Add8/1
  r_stat5/1 -> Multi3/1
  r_stat4/1 -> Multi2/1
  Multi1/1 -> Add6/1
  r_stat3/1 -> Multi1/1
  Bus Selector3/2 -> Add5/2  "<vl_RF>"
  Multi/1 -> Add5/1
  Bus Selector3/1 -> Multi/2  "<omega_RF>"
  Input/1 -> Bus Selector3/1, Bus Selector2/1
  Add5/1 -> Optimierung mit Lagrange Multiplikator Methode/4(vslip_FR)
  Add6/1 -> Optimierung mit Lagrange Multiplikator Methode/3(vslip_FL)
  r_stat2/1 -> Multi/1
  Optimierung mit Lagrange Multiplikator Methode/1(X_FL) -> Memory3/1, Limits berücksichtigen/11(X_FL), Scope2/4

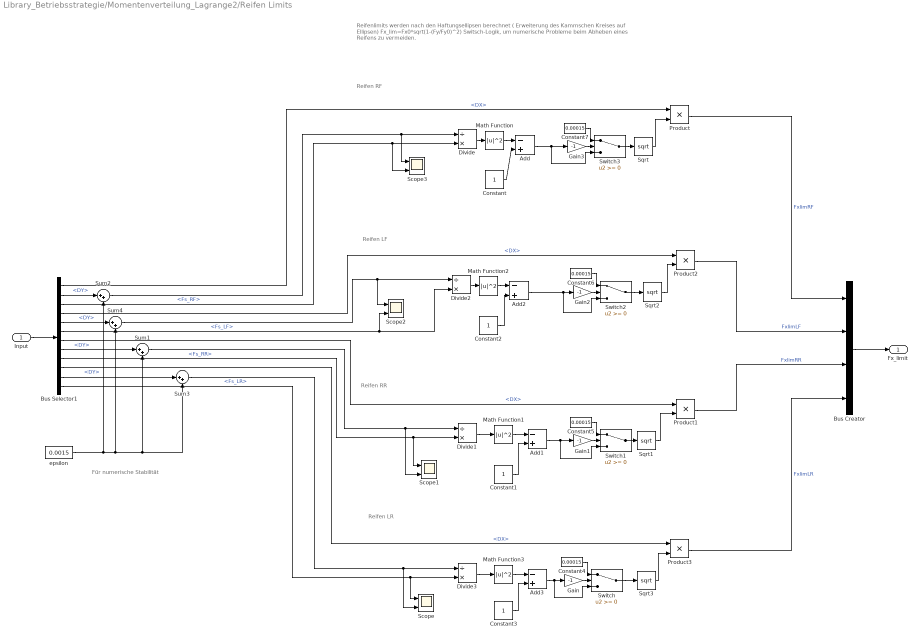
== system Library_Betriebsstrategie/Momentenverteilung_Lagrange2/Reifen Limits ==
  note: Reifenlimits werden nach den Haftungsellipsen berechnet ( Erweiterung des Kammschen Kreises auf Ellipsen)
      | Fx_lim=Fx0*sqrt(1-(Fy/Fy0)^2)
      |
      | Switsch-Logik, um numerische Probleme beim Abheben eines Reifens zu vermeiden.
  note: Für numerische Stabilität
  note: Reifen LR
  note: Reifen RR
  note: Reifen LF
  note: Reifen RF
  Input : Inport
  Add{,1..3} (4 alike) : Sum  Inputs=-+
  Bus Creator : BusCreator  Inputs=4
  Bus Selector1 : BusSelector  OutputSignals=F0.RF.DX,F0.RF.DY,Fs.Fs_RF,F0.LF.DX,F0.LF.DY,Fs.Fs_LF,F0.RR.DX,F0.RR.DY,Fs.Fs_RR,F0.LR.DX,F0.LR.DY,Fs.Fs_LR
  Constant{,1..3} (4 alike) : Constant
  Constant{4..7} (4 alike) : Constant  Value=0.00015
  Divide{,1..3} (4 alike) : Product  Inputs=/*
  Gain{,1..3} (4 alike) : Gain  Gain=-1
  Math Function{,1..3} (4 alike) : Math  Operator=magnitude^2  SaturateOnIntegerOverflow=on
  Product{,1..3} (4 alike) : Product
  Scope{,1..3} (4 alike) : Scope  NumInputPorts=2
  Sqrt{,1..3} (4 alike) : Sqrt  SaturateOnIntegerOverflow=on
  Sum{1..4} (4 alike) : Sum  Inputs=|++
  Switch{,1..3} (4 alike) : Switch
  epsilon : Constant  Value=0.0015
  Fx_limit : Outport
  wires:
  Switch3/1 -> Sqrt/1
  Constant7/1 -> Switch3/1
  Gain3/1 -> Switch3/2
  Add/1 -> Switch3/3, Gain3/1
  Switch2/1 -> Sqrt2/1
  Constant6/1 -> Switch2/1
  Gain2/1 -> Switch2/2
  Add2/1 -> Gain2/1, Switch2/3
  Switch1/1 -> Sqrt1/1
  Constant5/1 -> Switch1/1
  Gain1/1 -> Switch1/2
  Add1/1 -> Switch1/3, Gain1/1
  Switch/1 -> Sqrt3/1
  Constant4/1 -> Switch/1
  Gain/1 -> Switch/2
  Add3/1 -> Gain/1, Switch/3
  Bus Creator/1 -> Fx_limit/1
  Product3/1 -> Bus Creator/4  "FxlimLR"
  Product1/1 -> Bus Creator/3  "FxlimRR"
  Product2/1 -> Bus Creator/2  "FxlimLF"
  Product/1 -> Bus Creator/1  "FxlimRF"
  Bus Selector1/12 -> Scope/1, Divide3/2  "<Fs_LR>"
  Bus Selector1/9 -> Scope1/1, Divide1/2  "<Fs_RR>"
  Bus Selector1/6 -> Scope2/2, Divide2/2  "<Fs_LF>"
  Bus Selector1/3 -> Scope3/2, Divide/2  "<Fs_RF>"
  Input/1 -> Bus Selector1/1
  Divide/1 -> Math Function/1
  Sqrt3/1 -> Product3/2
  Constant3/1 -> Add3/2
  Math Function3/1 -> Add3/1
  Divide3/1 -> Math Function3/1
  Sum3/1 -> Scope/2, Divide3/1
  Sqrt2/1 -> Product2/2
  Constant2/1 -> Add2/2
  Math Function2/1 -> Add2/1
  Divide2/1 -> Math Function2/1
  Sum4/1 -> Scope2/1, Divide2/1
  Bus Selector1/4 -> Product2/1  "<DX>"
  Sqrt1/1 -> Product1/2
  Constant1/1 -> Add1/2
  Math Function1/1 -> Add1/1
  Divide1/1 -> Math Function1/1
  Sum1/1 -> Scope1/2, Divide1/1
  Bus Selector1/7 -> Product1/1  "<DX>"
  Sqrt/1 -> Product/2
  Constant/1 -> Add/2
  Math Function/1 -> Add/1
  Sum2/1 -> Scope3/1, Divide/1
  Bus Selector1/1 -> Product/1  "<DX>"
  epsilon/1 -> Sum2/2, Sum4/2, Sum1/2, Sum3/2
  Bus Selector1/2 -> Sum2/1  "<DY>"
  Bus Selector1/11 -> Sum3/1  "<DY>"
  Bus Selector1/8 -> Sum1/1  "<DY>"
  Bus Selector1/5 -> Sum4/1  "<DY>"
  Bus Selector1/10 -> Product3/1  "<DX>"

== system Library_Betriebsstrategie/Momentenverteilung_Regelbasiert/Feedback Controller ==
  note: 1/2 sigma(Tc)
  note: M_z punkt = - Iz * K * sign(sigma - 1/2sigma(Tc))
  note: Sigmoid Funktion
  Input : Inport
  Gierrate ref : Inport  Port=2
  -1 : Gain  Gain=-1
  Abs : Abs
  Add : Sum
  Bus Selector2 : BusSelector  OutputSignals=psi.psip
  Discrete D : simulink/Discrete/Discrete Derivative  gainval=1.0  ICPrevScaledInput=0.0  OutMin=[]  OutMax=[]  OutDataType=fixdt(1, 16)  OutScaling=2^-10  DoSatur=off
  Discrete-Time Integrator : DiscreteIntegrator  SampleTime=-1  ICPrevOutput=DiscIntNeverNeededParam  ICPrevScaledInput=DiscIntNeverNeededParam
  Divide : Product  Inputs=*/
  Divide1 : Product  Inputs=*/
  Einheitenkorrektur : Constant  Value=1000
  Gain : Gain  Gain=0.5
  K : Gain  Gain=8
  Memory : Memory  LinearizeAsDelay=on
  Product : Product
  Sum : Sum  Inputs=|-+
  Sum1 : Sum  Inputs=|+-
  Unit Delay : UnitDelay  SampleTime=-1
  Zero Crossing : Subsystem
  epsilon : Constant  Value=0.015
  M_z_desired : Outport
  wires:
  Gierrate ref/1 -> Sum/1
  Sum/1 -> Sum1/1, Zero Crossing/3(e0), Discrete D/1  "sigma = - error"
  Sum1/1 -> Divide/1, Abs/1
  Abs/1 -> Add/1
  epsilon/1 -> Add/2
  Add/1 -> Divide/2
  Divide/1 -> K/1
  K/1 -> Product/1
  Product/1 -> -1/1
  -1/1 -> Discrete-Time Integrator/1
  Discrete-Time Integrator/1 -> M_z_desired/1
  Discrete D/1 -> Zero Crossing/1(de0), Unit Delay/1
  Gain/1 -> Sum1/2
  Memory/1 -> Zero Crossing/4(e1)
  Unit Delay/1 -> Zero Crossing/2(de1)
  Zero Crossing/1(error(Tc)) -> Memory/1, Gain/1
  Einheitenkorrektur/1 -> Divide1/2
  Divide1/1 -> Product/2
  Input/1 -> Bus Selector2/1
  Bus Selector2/1 -> Sum/2  "<psip>"

== system Library_Betriebsstrategie/Momentenverteilung_Regelbasiert/Gierrate Referenz Berechnung ==
  note: Limit für die Gierrate
  note: Gewünschte Gierrate nach:
      | psip_desired = vx * delta / (l + vx^2 * K_us )
  input : Inport
  delta_wheel : Inport  Port=2
  2 Räder : Constant  Value=0.5
  Abs : Abs
  Abs1 : Abs
  Add : Sum
  Add1 : Sum  Inputs=+--
  Add2 : Sum
  Bus Selector1 : BusSelector  OutputSignals=delta_RF,delta_LF
  Bus Selector2 : BusSelector  OutputSignals=x.ax,beta.beta,beta.betap,x.vx
  Constant1 : Constant  Value=par_VEH.g
  Constant10 : Constant  Value=par_VEH.l
  Constant20 : Constant  Value=mu_road
  Divide : Product  Inputs=*/
  Divide1 : Product  Inputs=**/
  Divide2 : Product  Inputs=**/
  Divide3 : Product  Inputs=*/
  Kus : Constant  Value=0
  Product : Product
  Product1 : Product
  Product2 : Product
  Sicherheitsfaktor : Gain  Gain=0.90
  Sign : Signum
  Sqrt : Sqrt  SaturateOnIntegerOverflow=on
  Sum : Sum  Inputs=|++
  Sum1 : Sum  Inputs=|++
  delta mittel : Product
  eins : Constant
  epsilon : Constant  Value=0.0015
  min : MinMax  Inputs=2
  tan (beta)1 : Trigonometry  Operator=tan
  tan^2 (beta)1 : Math  Operator=square  SaturateOnIntegerOverflow=on
  vx^2 : Math  Operator=square  SaturateOnIntegerOverflow=on
  Gierrate ref : Outport
  wires:
  epsilon/1 -> Sum1/2
  Sum1/1 -> Divide1/3, Divide2/3
  Sqrt/1 -> Divide3/2
  Add2/1 -> Sqrt/1
  eins/1 -> Add2/2
  tan^2 (beta)1/1 -> Add2/1
  Bus Selector2/3 -> Divide3/1  "<betap>"
  Divide3/1 -> Add1/3
  Bus Selector2/2 -> tan (beta)1/1  "<beta>"
  tan (beta)1/1 -> Divide2/1, tan^2 (beta)1/1
  Bus Selector2/1 -> Divide2/2  "<ax>"
  Divide2/1 -> Add1/2
  Constant20/1 -> Divide1/1
  Constant1/1 -> Divide1/2
  Divide1/1 -> Add1/1
  Abs1/1 -> min/2
  Abs/1 -> min/1
  Product2/1 -> Gierrate ref/1
  min/1 -> Product2/2
  Sign/1 -> Product2/1  "Vorzeichen von delta"
  Add1/1 -> Sicherheitsfaktor/1
  Sicherheitsfaktor/1 -> Abs1/1  "Gierrate Limit"
  Bus Selector2/4 -> Product/1, vx^2/1, Sum1/1  "<vx>"
  input/1 -> Bus Selector2/1
  delta mittel/1 -> Product/2, Sign/1
  2 Räder/1 -> delta mittel/2
  Add/1 -> delta mittel/1
  Bus Selector1/2 -> Add/2  "<delta_LF>"
  Bus Selector1/1 -> Add/1  "<delta_RF>"
  delta_wheel/1 -> Bus Selector1/1
  Divide/1 -> Abs/1  "Gierrate gewuenscht"
  Kus/1 -> Product1/2
  Product1/1 -> Sum/1
  Sum/1 -> Divide/2
  vx^2/1 -> Product1/1
  Constant10/1 -> Sum/2
  Product/1 -> Divide/1

== system Library_Betriebsstrategie/Momentenverteilung_Regelbasiert/Limitierungen gesamt ==
  Fx_limit : Inport
  M_limit : Inport  Port=2
  Bus Creator : BusCreator  Inputs=8
  Bus Selector : BusSelector  OutputSignals=FxlimRF,FxlimLF,FxlimRR,FxlimLR
  Bus Selector1 : BusSelector  OutputSignals=M_RF_ub,M_RF_lb,M_LF_ub,M_LF_lb,M_RR_ub,M_RR_lb,M_LR_ub,M_LR_lb
  Divide{,1..7} (8 alike) : Product  Inputs=*/
  Gain{,1..3} (4 alike) : Gain  Gain=-1
  Max_FL : MinMax  Function=max  Inputs=2
  Max_FR : MinMax  Function=max  Inputs=2
  Max_FR1 : MinMax  Function=max  Inputs=2
  Max_RR : MinMax  Function=max  Inputs=2
  Min_FL : MinMax  Inputs=2
  Min_FR : MinMax  Inputs=2
  Min_FR1 : MinMax  Inputs=2
  Min_RR : MinMax  Inputs=2
  r_stat{0..7} (8 alike) : Constant  Value=par_VEH.r_stat0
  Fx_limits : Outport
  wires:
  Bus Selector/4 -> Min_FR1/1, Gain3/1  "<FxlimLR>"
  Bus Selector1/8 -> Divide7/1  "<M_LR_lb>"
  Bus Selector1/7 -> Divide6/1  "<M_LR_ub>"
  Max_FR1/1 -> Bus Creator/8  "Fx_RL_lb"
  Gain3/1 -> Max_FR1/1
  Divide7/1 -> Max_FR1/2
  r_stat7/1 -> Divide7/2
  Min_FR1/1 -> Bus Creator/7  "Fx_RL_ub"
  Divide6/1 -> Min_FR1/2
  r_stat6/1 -> Divide6/2
  Bus Selector/3 -> Min_RR/1, Gain2/1  "<FxlimRR>"
  Bus Selector1/6 -> Divide5/1  "<M_RR_lb>"
  Bus Selector1/5 -> Divide4/1  "<M_RR_ub>"
  Max_RR/1 -> Bus Creator/6  "Fx_RR_lb"
  Gain2/1 -> Max_RR/1
  Divide5/1 -> Max_RR/2
  r_stat5/1 -> Divide5/2
  Min_RR/1 -> Bus Creator/5  "Fx_RR_ub"
  Divide4/1 -> Min_RR/2
  r_stat4/1 -> Divide4/2
  Max_FL/1 -> Bus Creator/4  "Fx_FL_lb"
  Min_FL/1 -> Bus Creator/3  "Fx_FL_ub"
  Bus Selector1/4 -> Divide3/1  "<M_LF_lb>"
  Bus Selector1/3 -> Divide2/1  "<M_LF_ub>"
  Bus Selector/2 -> Min_FL/1, Gain1/1  "<FxlimLF>"
  Gain1/1 -> Max_FL/1
  Divide3/1 -> Max_FL/2
  r_stat3/1 -> Divide3/2
  Divide2/1 -> Min_FL/2
  r_stat2/1 -> Divide2/2
  Max_FR/1 -> Bus Creator/2  "Fx_FR_lb"
  Gain/1 -> Max_FR/1
  Divide1/1 -> Max_FR/2
  r_stat1/1 -> Divide1/2
  Bus Selector1/2 -> Divide1/1  "<M_RF_lb>"
  Min_FR/1 -> Bus Creator/1  "Fx_FR_ub"
  Bus Creator/1 -> Fx_limits/1
  Divide/1 -> Min_FR/2
  r_stat0/1 -> Divide/2
  Bus Selector/1 -> Min_FR/1, Gain/1  "<FxlimRF>"
  Bus Selector1/1 -> Divide/1  "<M_RF_ub>"
  M_limit/1 -> Bus Selector1/1
  Fx_limit/1 -> Bus Selector/1

== system Library_Betriebsstrategie/Momentenverteilung_Regelbasiert/Momente für die Reibbremse ==
  M_antr : Inport
  M_wheel : Inport  Port=2
  v_x : Inport  Port=3
  bkv : Inport  Port=4
  Add : Sum  Inputs=-+
  Add1 : Sum  Inputs=++++
  Bias : Bias  Bias=-1
  Bus Creator1 : BusCreator  Inputs=4
  Bus Selector : BusSelector  OutputSignals=M_antr_LF,M_antr_LR,M_antr_RF,M_antr_RR
  Product4 : Product  Inputs=3
  Product5 : Product  Inputs=3
  Saturation2 : Saturate  UpperLimit=0  LowerLimit=-5000
  Sign : Signum
  Signal Conversion : SignalConversion  OverrideOpt=off
  Signal Conversion1 : SignalConversion  OverrideOpt=off
  Unary Minus : UnaryMinus
  Unit Delay2 : UnitDelay  InitialCondition=2  SampleTime=-1
  M_brems : Outport
  wires:
  Add/1 -> Saturation2/1
  Saturation2/1 -> Product5/1, Product4/2
  Bias/1 -> Unary Minus/1
  Unary Minus/1 -> Product5/2
  Sign/1 -> Product4/3, Product5/3
  Unit Delay2/1 -> Sign/1
  bkv/1 -> Product4/1, Bias/1
  v_x/1 -> Unit Delay2/1
  M_wheel/1 -> Add/2
  M_antr/1 -> Bus Selector/1
  Bus Selector/4 -> Add1/4  "<M_antr_RR>"
  Bus Selector/3 -> Add1/3  "<M_antr_RF>"
  Bus Selector/2 -> Add1/2  "<M_antr_LR>"
  Bus Selector/1 -> Add1/1  "<M_antr_LF>"
  Add1/1 -> Add/1
  Bus Creator1/1 -> M_brems/1
  Product4/1 -> Bus Creator1/1, Signal Conversion/1  "M_brems_LF"
  Signal Conversion/1 -> Bus Creator1/2  "M_brems_LR"
  Product5/1 -> Signal Conversion1/1, Bus Creator1/3  "M_brems_RF"
  Signal Conversion1/1 -> Bus Creator1/4  "M_brems_RR"

== system Library_Betriebsstrategie/Momentenverteilung_Regelbasiert/Motor Limits ==
  Input : Inport
  Add{1..4} (4 alike) : Sum
  Bus Creator : BusCreator  Inputs=8
  Bus Selector : BusSelector  OutputSignals=omega
  Demux : Demux
  Demux1 : Demux
  Gain{,1..7} (8 alike) : Gain  Gain=0.5
  M_Antr : Lookup_n-D  NumberOfTableDimensions=1  BreakpointsForDimension1=par_VEH.dt_nmax/par_VEH.dt_i/60*2*pi  Table=par_VEH.dt_Mmax*par_VEH.dt_i/2  InternalRulePriority=Speed  RndMeth=Simplest  InputSameDT=on
  M_Reku : Lookup_n-D  NumberOfTableDimensions=1  BreakpointsForDimension1=par_VEH.dt_nmin/par_VEH.dt_i/60*2*pi  Table=par_VEH.dt_Mmin*par_VEH.dt_i/2  InternalRulePriority=Speed  RndMeth=Simplest  InputSameDT=on
  Rate Transition : RateTransition  OutPortSampleTime=stepsize*10
  Rate Transition1 : RateTransition  OutPortSampleTimeOpt=Inherit  OutPortSampleTime=0.001
  Rate Transition2 : RateTransition  OutPortSampleTime=stepsize*10
  Rate Transition3 : RateTransition  OutPortSampleTimeOpt=Inherit  OutPortSampleTime=0.001
  M_limit : Outport
  wires:
  Bus Creator/1 -> M_limit/1
  M_Reku/1 -> Rate Transition1/1
  Rate Transition/1 -> M_Reku/1
  M_Antr/1 -> Rate Transition3/1
  Rate Transition2/1 -> M_Antr/1
  Rate Transition1/1 -> Demux/1
  Demux/1 -> Add1/1
  Demux/2 -> Add1/2
  Add1/1 -> Gain4/1, Gain/1
  Demux/3 -> Add2/1
  Demux/4 -> Add2/2
  Add2/1 -> Gain5/1, Gain1/1
  Demux1/1 -> Add3/1
  Demux1/2 -> Add3/2
  Add3/1 -> Gain6/1, Gain2/1
  Demux1/3 -> Add4/1
  Demux1/4 -> Add4/2
  Add4/1 -> Gain7/1, Gain3/1
  Rate Transition3/1 -> Demux1/1
  Bus Selector/1 -> Rate Transition/1, Rate Transition2/1  "<omega>"
  Input/1 -> Bus Selector/1
  Gain1/1 -> Bus Creator/3  "M_RF_lb"
  Gain2/1 -> Bus Creator/5  "M_LF_ub"
  Gain3/1 -> Bus Creator/7  "M_RF_ub"
  Gain4/1 -> Bus Creator/1  "M_LF_lb"
  Gain/1 -> Bus Creator/2  "M_LR_lb"
  Gain5/1 -> Bus Creator/4  "M_RR_lb"
  Gain6/1 -> Bus Creator/6  "M_LR_ub"
  Gain7/1 -> Bus Creator/8  "M_RR_ub"

== system Library_Betriebsstrategie/Momentenverteilung_Regelbasiert/Radmomentenaufteilung ==
  Fx_limits : Inport
  Input : Inport  Port=2
  M_wheel : Inport  Port=3
  M_z_desired : Inport  Port=4
  Add{,1..3} (4 alike) : Sum
  Bus Creator : BusCreator  Inputs=4
  Bus Selector : BusSelector  OutputSignals=Fx_FR_ub,Fx_FL_ub,Fx_RR_ub,Fx_RL_ub
  Bus Selector1 : BusSelector  OutputSignals=Fz.Fz_RF,Fz.Fz_LF,Fz.Fz_RR,Fz.Fz_LR
  Divide : Product  Inputs=*/
  Divide1 : Product  Inputs=*/
  Optimale Verteilung : MATLAB Function  TreatAsAtomicUnit=on
  Product{,1..3} (4 alike) : Product
  Scope : Scope  NumInputPorts=4
  Scope1 : Scope  NumInputPorts=4
  epsilon : Constant  Value=0.0015
  r_stat{1..5} (5 alike) : Constant  Value=par_VEH.r_stat0
  sF05 : Constant  Value=(par_VEH.sF05 + par_VEH.sR05)*0.5
  M_antr : Outport
  wires:
  epsilon/1 -> Add3/2, Add2/2, Add1/2, Add/2
  Bus Selector1/4 -> Add3/1  "<Fz_LR>"
  Bus Selector1/3 -> Add2/1  "<Fz_RR>"
  Bus Selector1/2 -> Add1/1  "<Fz_LF>"
  Bus Selector1/1 -> Add/1  "<Fz_RF>"
  Add1/1 -> Optimale Verteilung/8(FzFL)
  Add2/1 -> Optimale Verteilung/9(FzRR)
  Add3/1 -> Optimale Verteilung/10(FzRL)
  Add/1 -> Optimale Verteilung/7(FzFR)
  r_stat5/1 -> Product3/2
  r_stat4/1 -> Product2/2
  r_stat3/1 -> Product1/2
  Optimale Verteilung/4(FxRL) -> Product3/1
  Optimale Verteilung/3(FxRR) -> Product2/1
  Optimale Verteilung/2(FxFL) -> Product1/1
  Product3/1 -> Bus Creator/4, Scope/1  "M_antr_LR"
  Product2/1 -> Bus Creator/3, Scope/2  "M_antr_RR"
  Product1/1 -> Bus Creator/2, Scope/3  "M_antr_LF"
  Product/1 -> Scope/4, Bus Creator/1  "M_antr_RF"
  Optimale Verteilung/1(FxFR) -> Product/1
  r_stat2/1 -> Product/2
  sF05/1 -> Divide1/2
  M_z_desired/1 -> Divide1/1
  Divide1/1 -> Optimale Verteilung/5(DeltaTV)
  Divide/1 -> Optimale Verteilung/6(DriverReq)
  r_stat1/1 -> Divide/2
  M_wheel/1 -> Divide/1
  Bus Creator/1 -> M_antr/1
  Fx_limits/1 -> Bus Selector/1
  Bus Selector/4 -> Optimale Verteilung/4(FxlimRL), Scope1/1  "<Fx_RL_ub>"
  Bus Selector/3 -> Optimale Verteilung/3(FxlimRR), Scope1/2  "<Fx_RR_ub>"
  Bus Selector/2 -> Optimale Verteilung/2(FxlimFL), Scope1/3  "<Fx_FL_ub>"
  Bus Selector/1 -> Optimale Verteilung/1(FxlimFR), Scope1/4  "<Fx_FR_ub>"
  Input/1 -> Bus Selector1/1

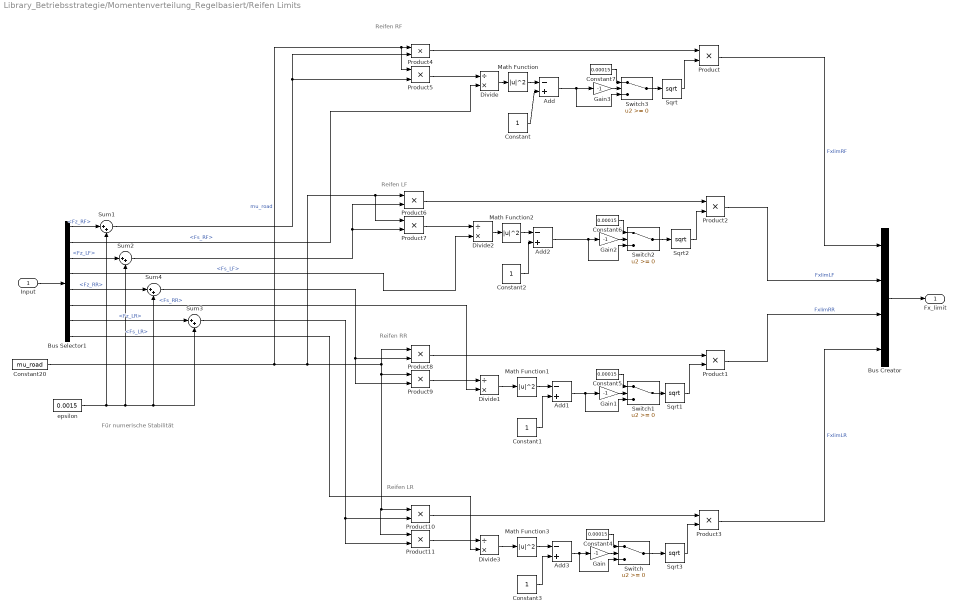
== system Library_Betriebsstrategie/Momentenverteilung_Regelbasiert/Reifen Limits ==
  note: Für numerische Stabilität
  note: Reifen LR
  note: Reifen RR
  note: Reifen LF
  note: Reifen RF
  Input : Inport
  Add{,1..3} (4 alike) : Sum  Inputs=-+
  Bus Creator : BusCreator  Inputs=4
  Bus Selector1 : BusSelector  OutputSignals=Fz.Fz_RF,Fs.Fs_RF,Fz.Fz_LF,Fs.Fs_LF,Fz.Fz_RR,Fs.Fs_RR,Fz.Fz_LR,Fs.Fs_LR
  Constant{,1..3} (4 alike) : Constant
  Constant20 : Constant  Value=mu_road
  Constant{4..7} (4 alike) : Constant  Value=0.00015
  Divide{,1..3} (4 alike) : Product  Inputs=/*
  Gain{,1..3} (4 alike) : Gain  Gain=-1
  Math Function{,1..3} (4 alike) : Math  Operator=magnitude^2  SaturateOnIntegerOverflow=on
  Product{,1..11} (12 alike) : Product
  Sqrt{,1..3} (4 alike) : Sqrt  SaturateOnIntegerOverflow=on
  Sum{1..4} (4 alike) : Sum  Inputs=|++
  Switch{,1..3} (4 alike) : Switch
  epsilon : Constant  Value=0.0015
  Fx_limit : Outport
  wires:
  Switch3/1 -> Sqrt/1
  Constant7/1 -> Switch3/1
  Gain3/1 -> Switch3/2
  Add/1 -> Switch3/3, Gain3/1
  Switch2/1 -> Sqrt2/1
  Constant6/1 -> Switch2/1
  Gain2/1 -> Switch2/2
  Add2/1 -> Gain2/1, Switch2/3
  Switch1/1 -> Sqrt1/1
  Constant5/1 -> Switch1/1
  Gain1/1 -> Switch1/2
  Add1/1 -> Switch1/3, Gain1/1
  Switch/1 -> Sqrt3/1
  Constant4/1 -> Switch/1
  Gain/1 -> Switch/2
  Add3/1 -> Gain/1, Switch/3
  Bus Creator/1 -> Fx_limit/1
  Product3/1 -> Bus Creator/4  "FxlimLR"
  Product1/1 -> Bus Creator/3  "FxlimRR"
  Product2/1 -> Bus Creator/2  "FxlimLF"
  Product/1 -> Bus Creator/1  "FxlimRF"
  Bus Selector1/8 -> Divide3/2  "<Fs_LR>"
  Bus Selector1/6 -> Divide1/2  "<Fs_RR>"
  Bus Selector1/4 -> Divide2/2  "<Fs_LF>"
  Bus Selector1/2 -> Divide/2  "<Fs_RF>"
  Constant20/1 -> Product5/1, Product4/1, Product6/1, Product7/1, Product10/1, Product11/1, Product9/1, Product8/1  "mu_road"
  Input/1 -> Bus Selector1/1
  Divide/1 -> Math Function/1
  Sqrt3/1 -> Product3/2
  Constant3/1 -> Add3/2
  Math Function3/1 -> Add3/1
  Divide3/1 -> Math Function3/1
  Product11/1 -> Divide3/1
  Product10/1 -> Product3/1
  Sqrt2/1 -> Product2/2
  Constant2/1 -> Add2/2
  Math Function2/1 -> Add2/1
  Divide2/1 -> Math Function2/1
  Product7/1 -> Divide2/1
  Product6/1 -> Product2/1
  Sqrt1/1 -> Product1/2
  Constant1/1 -> Add1/2
  Math Function1/1 -> Add1/1
  Divide1/1 -> Math Function1/1
  Product9/1 -> Divide1/1
  Product8/1 -> Product1/1
  Sqrt/1 -> Product/2
  Constant/1 -> Add/2
  Math Function/1 -> Add/1
  Product5/1 -> Divide/1
  Product4/1 -> Product/1
  Bus Selector1/1 -> Sum1/1  "<Fz_RF>"
  Sum1/1 -> Product4/2, Product5/2
  Bus Selector1/3 -> Sum2/1  "<Fz_LF>"
  Sum2/1 -> Product7/2, Product6/2
  Bus Selector1/5 -> Sum4/1  "<Fz_RR>"
  Sum4/1 -> Product9/2, Product8/2
  Bus Selector1/7 -> Sum3/1  "<Fz_LR>"
  Sum3/1 -> Product10/2, Product11/2
  epsilon/1 -> Sum1/2, Sum3/2, Sum4/2, Sum2/2

== system Library_Betriebsstrategie/Momentverteilung_LR/Feedback Controller ==
  note: 1/2 sigma(Tc)
  note: M_z punkt = - Iz * K * sign(sigma - 1/2sigma(Tc))
  note: Sigmoid Funktion
  Gierrate : Inport
  Gierrate ref : Inport  Port=2
  Iz : Inport  Port=3
  -1 : Gain  Gain=-1
  Abs : Abs
  Add : Sum
  Discrete D : simulink/Discrete/Discrete Derivative  gainval=1.0  ICPrevScaledInput=0.0  OutMin=[]  OutMax=[]  OutDataType=fixdt(1, 16)  OutScaling=2^-10  DoSatur=off
  Discrete-Time Integrator : DiscreteIntegrator  SampleTime=0.1  ICPrevOutput=DiscIntNeverNeededParam  ICPrevScaledInput=DiscIntNeverNeededParam
  Divide : Product  Inputs=*/
  Divide1 : Product  Inputs=*/
  Einheitenkorrektur : Constant  Value=1000
  Gain : Gain  Gain=0.5
  K : Gain  Gain=8
  Memory : Memory  LinearizeAsDelay=on
  Product : Product
  Sum : Sum  Inputs=|-+
  Sum1 : Sum  Inputs=|+-
  Unit Delay : UnitDelay  SampleTime=0.1
  Zero Crossing : Subsystem
  epsilon : Constant  Value=0.015
  M_z_desired : Outport
  wires:
  Gierrate/1 -> Sum/2
  Gierrate ref/1 -> Sum/1
  Sum/1 -> Sum1/1, Zero Crossing/3(e0), Discrete D/1  "sigma = - error"
  Sum1/1 -> Divide/1, Abs/1
  Abs/1 -> Add/1
  epsilon/1 -> Add/2
  Add/1 -> Divide/2
  Divide/1 -> K/1
  K/1 -> Product/1
  Product/1 -> -1/1
  -1/1 -> Discrete-Time Integrator/1
  Discrete-Time Integrator/1 -> M_z_desired/1
  Discrete D/1 -> Zero Crossing/1(de0), Unit Delay/1
  Gain/1 -> Sum1/2
  Memory/1 -> Zero Crossing/4(e1)
  Unit Delay/1 -> Zero Crossing/2(de1)
  Zero Crossing/1(error(Tc)) -> Memory/1, Gain/1
  Iz/1 -> Divide1/1
  Einheitenkorrektur/1 -> Divide1/2
  Divide1/1 -> Product/2
